simulink model "torque_in"  (R2017a)
settings: Solver=VariableStepAuto  StartTime=0.0  StopTime=10.0  RelTol=1e-3
settings Model: Creator=nathaniel  LastModifiedBy=nathaniel

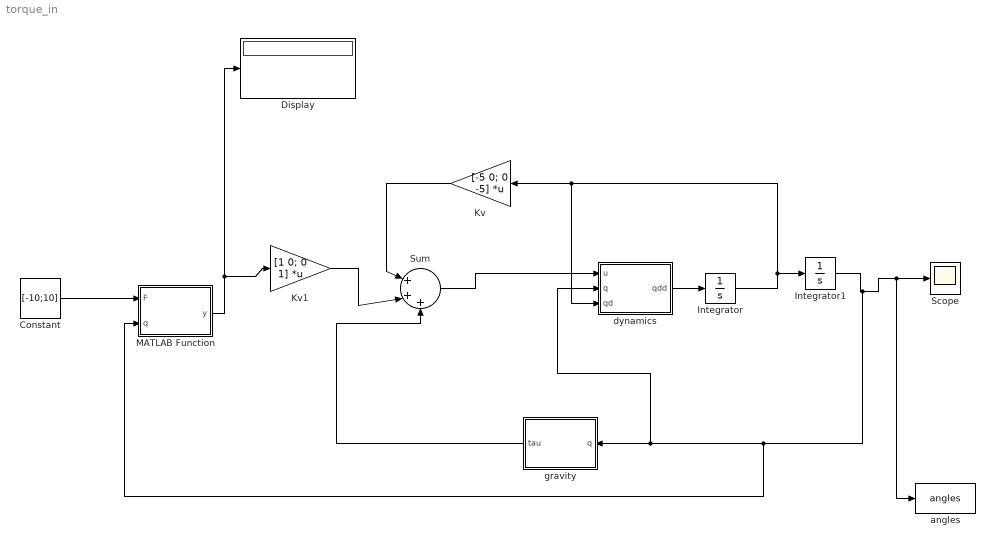
== system torque_in ==
  Constant : Constant  Value=[-10;10]  VectorParams1D=off
  Display : Display
  Integrator : Integrator  InitialCondition=[0;0]  ContinuousStateAttributes='vel'
  Integrator1 : Integrator  InitialCondition=[0;0]  ZeroCross=off  ContinuousStateAttributes='pos'
  Kv : Gain  Gain=[-5 0; 0 -5]  Multiplication=Matrix(K*u) (u vector)
  Kv1 : Gain  Gain=[1 0; 0 1]  Multiplication=Matrix(K*u) (u vector)
  MATLAB Function : MATLAB Function  TreatAsAtomicUnit=on
  Scope : Scope
  Sum : Sum  Inputs=|+++
  angles : ToWorkspace  VariableName=angles  SampleTime=-1
  dynamics : MATLAB Function  TreatAsAtomicUnit=on
  gravity : MATLAB Function  TreatAsAtomicUnit=on
  wires:
  dynamics/1(qdd) -> Integrator/1
  gravity/1(tau) -> Sum/3
  Kv/1 -> Sum/1
  Sum/1 -> dynamics/1(u)
  Integrator1/1 -> MATLAB Function/2(q), dynamics/2(q), gravity/1(q), angles/1, Scope/1
  Integrator/1 -> dynamics/3(qd), Kv/1, Integrator1/1
  Constant/1 -> MATLAB Function/1(F)
  MATLAB Function/1(y) -> Kv1/1, Display/1
  Kv1/1 -> Sum/2

== matlab function torque_in/MATLAB Function ==
  data: F input; y output; q input
function y = fcn(F,q)

l1 = 1;
l2 = 1;
J = [ -l1*sin(q(1)) - l2*sin(sum(q)), l1*cos(q(1)) + l2*cos(sum(q));
      -l2*sin(sum(q)), l2*cos(sum(q))];
 
y = J*F;
end

== matlab function torque_in/gravity ==
  data: q input; tau output
function tau = fcn(q)

tau = gravity(q);
end

== matlab function torque_in/dynamics ==
  data: u input; qdd output; q input; qd input
function qdd = fcn(u,q,qd)

qdd = dynamics(u,q,qd);
